simulink model "V.1.0.SystemsmModelling"  (R2020a)
settings: Solver=ode23t  StartTime=0.0  StopTime=2000  MaxStep=2000.0  RelTol=1e-3
values from neighbouring files (symbols this model uses):
  InitialTemp = 300    [Setup.m]
undefined symbols (not defined in the file or in its folder): commanded_mass_flow, compressor_time_constant, condenser_length, copper_density, environment_temperature, evaporator_length, ground_temperature, max_throat_area, max_throat_temperature, min_throat_area, min_throat_temperature, pipe_diameter, pipe_thickness, target_temperature, temperature_delta, u_sat
libraries: fl_lib x208, refrigeration_lib x90, fl_ps_legacy_lib x50, nesl_utility x45
(part 1 of 7)
settings Model: Creator=denni  LastModifiedBy=denni

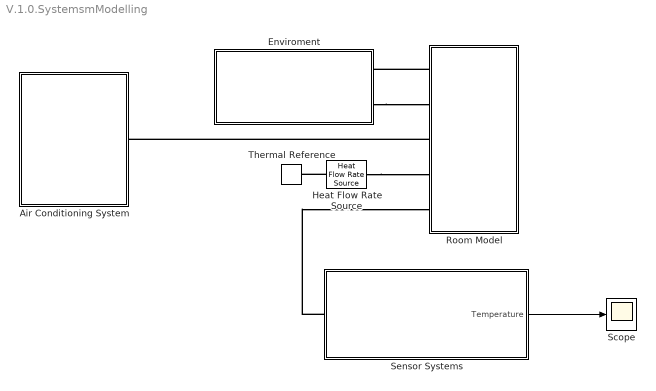
== system V.1.0.SystemsmModelling ==
  Air Conditioning System : Subsystem
  Enviroment : Subsystem
  Heat Flow Rate Source : fl_lib/Thermal/Thermal Sources/Heat Flow Rate Source  heat_flow=10 W
      settings: SourceProductBaseCode=SS  InternalSimscapePortConfiguration="{\"Bottom\":[],\"Left\":[{\"id\":\"B\",\"label\":\"B\",\"type\":\"foundation.thermal.thermal\"}],\"Right\":[{\"id\":\"A\",\"label\":\"A\",\"type\":\"foundation.thermal.thermal\"}],\"Top\":[]}"
  Room Model : Subsystem
  Scope : Scope
  Sensor Systems : Subsystem
  Thermal Reference : fl_lib/Thermal/Thermal Elements/Thermal Reference
  wires:
  Sensor Systems/1("Temperature ") -> Scope/1
  connections:
  Room Model/LConn1 -- Enviroment/LConn1
  Enviroment/LConn2 -- Room Model/LConn2
  Sensor Systems/LConn1 -- Room Model/LConn5
  Heat Flow Rate Source/LConn1 -- Room Model/LConn4
  Heat Flow Rate Source/RConn1 -- Thermal Reference/LConn1
  Room Model/LConn3 -- Air Conditioning System/RConn1

== system V.1.0.SystemsmModelling/Air Conditioning System ==
  Air Conditioner Model : Subsystem
  Air Conditioner Model1 : Subsystem
  Air Conditioner Model2 : Subsystem
  Air Conditioner Model3 : Subsystem
  Air Conditioner Model4 : Subsystem
  Air Conditioner Model5 : Subsystem
  Air Conditioner Model6 : Subsystem
  Air Conditioner Model7 : Subsystem
  Air Conditioner Model8 : Subsystem
  Air Conditioner Model9 : Subsystem
  Air : PMIOPort  Side=Right
  connections:
  Air Conditioner Model/LConn1 -- Air/RConn1 -- Air Conditioner Model1/LConn1 -- Air Conditioner Model2/LConn1 -- Air Conditioner Model5/LConn1 -- Air Conditioner Model8/LConn1 -- Air Conditioner Model9/LConn1 -- Air Conditioner Model7/LConn1 -- Air Conditioner Model6/LConn1 -- Air Conditioner Model4/LConn1 -- Air Conditioner Model3/LConn1

== system V.1.0.SystemsmModelling/Enviroment ==
  Atm Temperature Source : fl_lib/Thermal/Thermal Sources/Controlled Temperature Source
  Constant : Constant  Value=environment_temperature
  Constant1 : Constant  Value=ground_temperature
  Ground Temperature Source : fl_lib/Thermal/Thermal Sources/Controlled Temperature Source
  Simulink-PS Converter : nesl_utility/Simulink-PS Converter  PhysicalDomain=network_engine_domain  SubClassName=ps_input  LeftPortType=input  RightPortType=output  PseudoPeriodic=off  Frequencies=[]  NoiseDistribution=none  NoiseParameters=[]  Unit=1  AffineConversion=off  FilteringAndDerivatives=provide  SimscapeFilterOrder=1  InputFilterTimeConstant=0.001  UdotUserProvided=0
  Simulink-PS Converter1 : nesl_utility/Simulink-PS Converter  PhysicalDomain=network_engine_domain  SubClassName=ps_input  LeftPortType=input  RightPortType=output  PseudoPeriodic=off  Frequencies=[]  NoiseDistribution=none  NoiseParameters=[]  Unit=1  AffineConversion=off  FilteringAndDerivatives=provide  SimscapeFilterOrder=1  InputFilterTimeConstant=0.001  UdotUserProvided=0
  Thermal Reference1 : fl_lib/Thermal/Thermal Elements/Thermal Reference
  Thermal Reference2 : fl_lib/Thermal/Thermal Elements/Thermal Reference
  Atm Temperature Source1 : PMIOPort  Side=Left
  Ground Temperature Source1 : PMIOPort  Port=2  Side=Left
  wires:
  Constant/1 -> Simulink-PS Converter/1
  Constant1/1 -> Simulink-PS Converter1/1
  connections:
  Thermal Reference2/LConn1 -- Ground Temperature Source/RConn2
  Thermal Reference1/LConn1 -- Atm Temperature Source/RConn2
  Simulink-PS Converter1/RConn1 -- Ground Temperature Source/RConn1
  Ground Temperature Source/LConn1 -- Ground Temperature Source1/RConn1
  Atm Temperature Source1/RConn1 -- Atm Temperature Source/LConn1
  Simulink-PS Converter/RConn1 -- Atm Temperature Source/RConn1

== system V.1.0.SystemsmModelling/Room Model ==
  "Room Element " : Subsystem
  Solver Configuration : nesl_utility/Solver Configuration  PhysicalDomain=network_engine_domain  SubClassName=solver  LeftPortType=input  RightPortType=generic  Tones=[]  Harmonics=[]  SimulateNoise=off  Profile=off  UseLocalSampling=off  EnableSwitchedLinearOptims=on  FrequencyDomain=off  UseCCode=off  RelTol=0.001  AbsTol=1e-06  MinStep=1e-09  ToWorkspace=off  RevertToSquareIcSolve=off  NumHomotopyIterations=100  PhasorMode=off  PhasorModeNumHarmonics=1  DoDC=off  ResidualTolerance=1e-09  UseLocalSolver=off  LocalSolverChoice=NE_BACKWARD_EULER_ADVANCER  LocalSolverSampleTime=0.001  DoFixedCost=off  MaxNonlinIter=3  MaxModeIter=2  LinearAlgebra=auto  EquationFormulation=NE_TIME_EF  DelaysMemoryBudget=1024  AutomaticFiltering=on  FilteringTimeConstant=0.001  PartitionStorageMethod=AS_NEEDED  PartitionMemoryBudget=1024  PartitionMethod=ROBUST
  Thermal Mass Air : fl_lib/Thermal/Thermal Elements/Thermal Mass  mass=1 kg  sp_heat=1012 J/kg/K  T_specify=off  T_priority=High  T=300 K  T_nominal_specify=off  T_nominal_unit=K  T_nominal_value=1  Q_specify=off  Q_priority=None  Q=0 W  Q_nominal_specify=off  Q_nominal_unit=W  Q_nominal_value=1
  Atm-env : PMIOPort  Side=Left
  Ground-env : PMIOPort  Port=2  Side=Left
  Air Conditioner : PMIOPort  Port=3  Side=Left
  Server Racks : PMIOPort  Port=4  Side=Left
  "Room Temperature Sensor " : PMIOPort  Port=5  Side=Left
  connections:
  Thermal Mass Air/LConn1 -- Server Racks/RConn1 -- Air Conditioner/RConn1 -- "Room Temperature Sensor "/RConn1 -- Solver Configuration/RConn1 -- "Room Element "/LConn1
  Atm-env/RConn1 -- "Room Element "/LConn2
  "Room Element "/LConn3 -- Ground-env/RConn1

== system V.1.0.SystemsmModelling/Sensor Systems ==
  PS-Simulink Converter : nesl_utility/PS-Simulink Converter  PhysicalDomain=network_engine_domain  SubClassName=ps_output  LeftPortType=input  RightPortType=output  PseudoPeriodic=off  Frequencies=[]  Unit=inherit  AffineConversion=off
  Room Temperature Sensor : fl_lib/Thermal/Thermal Sensors/Temperature Sensor
  Thermal Reference : fl_lib/Thermal/Thermal Elements/Thermal Reference
  Room Temperature Sensor1 : PMIOPort  Side=Left
  "Temperature " : Outport
  wires:
  PS-Simulink Converter/1 -> "Temperature "/1
  connections:
  PS-Simulink Converter/LConn1 -- Room Temperature Sensor/RConn2
  Thermal Reference/LConn1 -- Room Temperature Sensor/RConn1
  Room Temperature Sensor/LConn1 -- Room Temperature Sensor1/RConn1

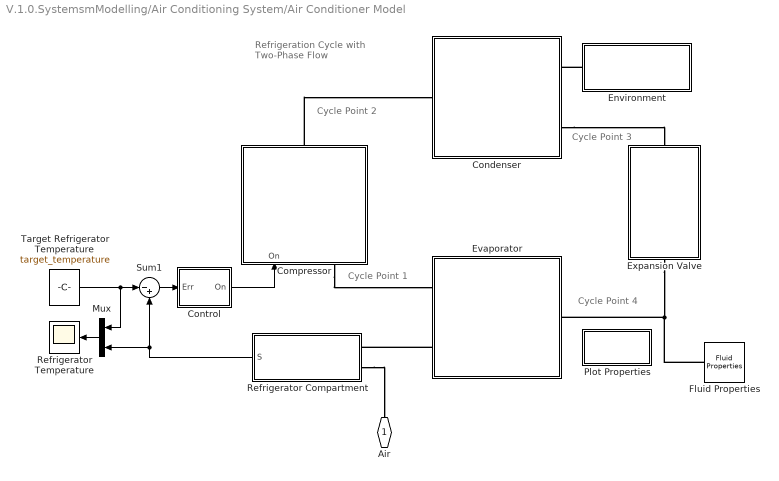
== system V.1.0.SystemsmModelling/Air Conditioning System/Air Conditioner Model ==
  note: Refrigeration Cycle
      | with Two-Phase Flow
  note: Cycle Point 1
  note: Cycle Point 3
  note: Cycle Point 2
  note: Cycle Point 4
  Compressor : Subsystem
      mask Display:
      | % Fading color
      | % Center to right
      | patch(sin(0.00*pi:0.05:1.10*pi),cos(0.00*pi:0.05:1.10*pi),[1;0.90;0.94]);
      | patch(sin(0.05*pi:0.05:0.95*pi),cos(0.05*pi:0.05:0.95*pi),[1;0.85;0.88]);
      | patch(sin(0.10*pi:0.05:0.90*pi),cos(0.10*pi:0.05:0.90*pi),[1;0.80;0.82]);
      | patch(sin(0.15*pi:0.05:0.85*pi),cos(0.15*pi:0.05:0.85*pi),[1;0.75;0.76]);
      | patch(sin(0.20*pi:0.05:0.80*pi),cos(0.20*pi:0.05:0.80*pi),[1;0.70;0.70]);
      | % Center to left
      | patch(sin(1.00*pi:0.05:2.00*pi),cos(1.00*pi:0.05:2.00*pi),[0.94;0.90;1]);
      | patch(sin(1.05*pi:0.05:1.95*pi),cos(1.05*pi:0.05:1.95*pi),[0.88;0.90;1]);
      | patch(sin(1.10*pi:0.05:1.90*pi),cos(1.10*pi:0.05:1.90*pi),[0.82;0.90;1]);
      | patch(sin(1.15*pi:0.05:1.85*pi),cos(1.15*pi:0.05:1.85*pi),[0.76;0.90;1]);
      | patch(sin(1.20*pi:0.05:1.80*pi),cos(1.20*pi:0.05:1.80*pi),[0.70;0.90;1]);
      | % Circle
      | plot(sin(0:0.1:2.2*pi),cos(0:0.1:2.2*pi));
      | % Angled lines
      | plot(sin([-0.6*pi/3 3.6*pi/8]),cos([-0.6*pi/3 3.6*pi/8]));
      | plot(sin([-0.6*pi/3 3.6*pi/8]),-cos([-0.6*pi/3 3.6*pi/8]));
      | plot(1.15*sin([-pi/4 3*pi/4]),1.15*cos([-pi/4 3*pi/4]));
      | % Arrow
      | patch([1.15*sin(-pi/4)+0.01;1.15*sin(3*pi/4)+0.01;1.15*sin(3*pi/4)-0.01;1.15*sin(-pi/4)-0.01],[1.15*cos(-pi/4)+0.01;1.15*cos(3*pi/4)+0.01;1.15*cos(3*pi/4)-0.01;1.15*cos(-pi/4)-0.01],[0;0;0])
      | patch([0.8*sin(3*pi/4)+0.05;1.15*sin(3*pi/4)+0.00;1.15*sin(3*pi/4)-0.00;0.8*sin(3*pi/4)-0.05],[0.8*cos(3*pi/4)+0.05;1.15*cos(3*pi/4)+0.00;1.15*cos(3*pi/4)-0.00;0.8*cos(3*pi/4)-0.05],[0;0;0])
      | % Points to set range for plotting area
      | color('white');plot(1.3,1.3);plot(-1.3,-1.3)
      | color('black');
      | 
      | port_label('LConn',1,'A');
      | port_label('RConn',1,'B');
      | port_label('input',1,'On');
  Condenser : Subsystem
      mask Display:
      | % Colored patches
      | % Center to right
      | patch(sin(0.0*pi:0.05:1.1*pi),cos(0.0*pi:0.05:1.1*pi),[1;0.58;0.58]);
      | patch(sin(0.1*pi:0.05:0.9*pi),cos(0.1*pi:0.05:0.9*pi),[1;0.64;0.64]);
      | patch(sin(0.2*pi:0.05:0.8*pi),cos(0.2*pi:0.05:0.8*pi),[1;0.70;0.70]);
      | % Center to left
      | patch(sin(1.0*pi:0.05:2.0*pi),cos(1.0*pi:0.05:2.0*pi),[1;0.52;0.52]);
      | patch(sin(1.1*pi:0.05:1.9*pi),cos(1.1*pi:0.05:1.9*pi),[1;0.46;0.46]);
      | patch(sin(1.2*pi:0.05:1.8*pi),cos(1.2*pi:0.05:1.8*pi),[1;0.40;0.40]);
      | % Circle
      | plot(sin(0:0.1:2.2*pi),cos(0:0.1:2.2*pi));
      | % 'M'
      | plot([0.5 0.5],[-1.2 0.5]);
      | plot([-0.5 -0.5],[-1.2 0.5]);
      | plot([0.5 0],[0.5 -0.2]);
      | plot([-0.5 0],[0.5 -0.2]);
      | % Plot points to set plot range
      | color('white');plot(1.3,1.3);plot(-1.3,-1.3)
      | color('black');
      | 
      | port_label('RConn',1,'A');
      | port_label('LConn',1,'T');
      | port_label('LConn',2,'B');
  Control : Subsystem
  Environment : Subsystem
      mask Display:
      | % Colored patch
      | patch([sin(0:0.1:1*pi)*0.25+0.4 sin(pi:0.1:2*pi)*0.25-0.4],[cos(0:0.1:1*pi) cos(pi:0.1:2*pi)],[1;0.9;0.9]);
      | % Outer rounded rectangle
      | plot(sin(0:0.1:1*pi)*0.25+0.4,cos(0:0.1:1*pi));
      | plot(sin(pi:0.1:2*pi)*0.25-0.4,cos(pi:0.1:2*pi));
      | plot([-0.4 0.4],[1 1]);
      | plot([-0.4 0.4],[-1 -1]);
      | % House frame
      | plot([-0.3 -0.3],[-0.866,0.866*0.2])
      | plot([0.3 0.3],[-0.866,0.866*0.2])
      | plot([0.3 0],[0.866*0.2, 0.866])
      | plot([-0.3 0],[0.866*0.2, 0.866])
      | plot([-0.3 0.3],[-0.866 -0.866])
      | plot([-0.3 0.3],[0.866 0.866]*0.2)
      | plot([-0.2 -0.04],[0.866 0.866]*0)
      | % Window
      | plot([-0.2 -0.04],[-1 -1]*0.2)
      | plot([-0.2 -0.04],[-1 -1]*0.4)
      | plot([-0.2 -0.2],[0 -0.4])
      | plot([-0.12 -0.12],[0 -0.4])
      | plot([-0.04 -0.04],[0 -0.4])
      | % Door
      | plot([0.05 0.05],[-0.866 -0.2])
      | plot([0.18 0.18],[-0.866 -0.2])
      | plot([0.05 0.18],[-0.2 -0.2])
      | patch([0.12 0.15 0.12 0.15],[-0.5 -0.5 -0.54 -0.54],[0;0;0])
      | % Outer boundary (so plot labels are visible)
      | color('white');plot(0.8660,0.8660);plot(-0.8660,-0.8660)
      | color('black');
      | port_label('LConn',1,'T');
  Evaporator : Subsystem
      mask Display:
      | % Fading color
      | % Center to right
      | patch(sin(0.00*pi:0.05:1.10*pi),cos(0.00*pi:0.05:1.10*pi),[0.58;0.70;1]);
      | patch(sin(0.05*pi:0.05:0.95*pi),cos(0.05*pi:0.05:0.95*pi),[0.63;0.75;1]);
      | patch(sin(0.10*pi:0.05:0.90*pi),cos(0.10*pi:0.05:0.90*pi),[0.66;0.80;1]);
      | patch(sin(0.15*pi:0.05:0.85*pi),cos(0.15*pi:0.05:0.85*pi),[0.69;0.85;1]);
      | patch(sin(0.20*pi:0.05:0.80*pi),cos(0.20*pi:0.05:0.80*pi),[0.70;0.90;1]);
      | % Center to left
      | patch(sin(1.00*pi:0.05:2.00*pi),cos(1.00*pi:0.05:2.00*pi),[0.52;0.60;1]);
      | patch(sin(1.05*pi:0.05:1.95*pi),cos(1.05*pi:0.05:1.95*pi),[0.49;0.55;1]);
      | patch(sin(1.10*pi:0.05:1.90*pi),cos(1.10*pi:0.05:1.90*pi),[0.46;0.50;1]);
      | patch(sin(1.15*pi:0.05:1.85*pi),cos(1.15*pi:0.05:1.85*pi),[0.43;0.45;1]);
      | patch(sin(1.20*pi:0.05:1.80*pi),cos(1.20*pi:0.05:1.80*pi),[0.40;0.40;1]);
      | % Circle
      | plot(sin(0:0.1:2.2*pi),cos(0:0.1:2.2*pi));
      | % 'M'
      | plot([0.5 0.5],[-1.2 0.5]);
      | plot([-0.5 -0.5],[-1.2 0.5]);
      | plot([0.5 0],[0.5 -0.2]);
      | plot([-0.5 0],[0.5 -0.2]);
      | % Plot points to set plotting range
      | color('white');plot(1.3,1.3);plot(-1.3,-1.3)
      | color('black');
      | 
      | port_label('LConn',1,'A');
      | port_label('RConn',1,'B');
      | port_label('RConn',2,'T');
  Expansion Valve : Subsystem
      mask Display:
      | % Colored patches
      | patch([-1 -1 0],[0.5 -0.5 0],[1;0.4;0.4]);
      | patch([1 1 0],[0.5 -0.5 0],[0.4;0.4;1]);
      | % Valve
      | plot([1 1],[0.5 -0.5]);
      | plot([-1 -1],[0.5 -0.5]);
      | plot([-1 1],[0.5 -0.5]);
      | plot([-1 1],[-0.5 0.5]);
      | % Arrow
      | patch([1.15*sin(-pi/4-0.01);1.15*sin(-pi/4+0.01);1*sin(3*pi/4-0.01);1*sin(3*pi/4+0.01)],[1.15*cos(-pi/4-0.01);1.15*cos(-pi/4+0.01);1*cos(3*pi/4-0.01);1*cos(3*pi/4+0.01)],[0;0;0])
      | patch([0.8*sin(3*pi/4+0.07);1.15*sin(3*pi/4+0.00);1.15*sin(3*pi/4-0.00);0.8*sin(3*pi/4-0.07)],[0.8*cos(3*pi/4+0.07);1.15*cos(3*pi/4+0.00);1.15*cos(3*pi/4-0.00);0.8*cos(3*pi/4-0.07)],[0;0;0])
      | % Plot outer points to set plot range
      | color('white'); plot(-1.3,0); plot(1.3,0);
      | color('black');
      | port_label('LConn',1,'A');
      | port_label('RConn',1,'B');
  Fluid Properties : refrigeration_lib/Fluid Properties  p_TLU=p_TLU MPa  u_TLU=u_TLU kJ/kg  v_TLU=v_TLU m^3/kg  T_TLU=T_TLU K  mu_TLU=mu_TLU s*uPa  k_TLU=k_TLU W/(m*K)  Pr_TLU=Pr_TLU  u_liq=u_sat(:,1) kJ/kg  u_vap=u_sat(:,2) kJ/kg
      settings: InternalSimscapePortConfiguration="{\"Bottom\":[],\"Left\":[],\"Right\":[{\"id\":\"A\",\"label\":\"\",\"type\":\"refrigeration.refrigeration\"}],\"Top\":[]}"
  Mux : Mux  Inputs=2
  Plot Properties : Subsystem
      settings: OpenFcn=plotFluidProperties()
      mask Display: disp('Plot Fluid\nProperties');
  Refrigerator Compartment : Subsystem
      mask Display:
      | % Color
      | patch([sin(0:0.1:1*pi)*0.25+0.4 sin(pi:0.1:2*pi)*0.25-0.4],[cos(0:0.1:1*pi) cos(pi:0.1:2*pi)],[0.70;0.90;1]);
      | % Outer rounded rectangle
      | plot(sin(pi:0.1:2*pi)*0.25-0.4,cos(pi:0.1:2*pi));
      | plot(sin(0:0.1:1*pi)*0.25+0.4,cos(0:0.1:1*pi));
      | plot(sin(pi:0.1:2*pi)*0.25-0.4,cos(pi:0.1:2*pi));
      | plot([-0.4 0.4],[1 1]);
      | plot([-0.4 0.4],[-1 -1]);
      | % Outer points to set size of plot range
      | color('white');plot(0.8660,0.8660);plot(-0.8660,-0.8660)
      | color('black');
      | % Snowflake
      | plot([0 0],[0.8 -0.8]);
      | plot([0 0.1],[0.5 0.7]);
      | plot([0 -0.1],[0.5 0.7]);
      | plot([0 0.1],[-0.5 -0.7]);
      | plot([0 -0.1],[-0.5 -0.7]);
      | plot(0.3*sin([pi/3 4*pi/3]),1*cos([pi/3 4*pi/3]));
      | plot([0.22*sin(pi/3) 0.25*sin(pi/4)],[0.7*cos(pi/3) 0.84*cos(pi/4)]);
      | plot([0.22*sin(pi/3) 0.25*sin(pi/2)],[0.7*cos(pi/3) 0.325*cos(pi/4)]);
      | plot([0.22*sin(pi/3) 0.25*sin(pi/4)],[-0.7*cos(pi/3) -0.84*cos(pi/4)]);
      | plot([0.22*sin(pi/3) 0.25*sin(pi/2)],[-0.7*cos(pi/3) -0.325*cos(pi/4)]);
      | plot(-0.3*sin([pi/3 4*pi/3]),1*cos([pi/3 4*pi/3]));
      | plot([-0.22*sin(pi/3) -0.25*sin(pi/4)],[0.7*cos(pi/3) 0.84*cos(pi/4)]);
      | plot([-0.22*sin(pi/3) -0.25*sin(pi/2)],[0.7*cos(pi/3) 0.325*cos(pi/4)]);
      | plot([-0.22*sin(pi/3) -0.25*sin(pi/4)],[-0.7*cos(pi/3) -0.84*cos(pi/4)]);
      | plot([-0.22*sin(pi/3) -0.25*sin(pi/2)],[-0.7*cos(pi/3) -0.325*cos(pi/4)]);
      | plot([0 0.1],[-0.5 -0.7]);
      | plot([0 -0.1],[-0.5 -0.7]);
      | % Labels
      | port_label('LConn',1,'T');
      | port_label('output',1,'S');
  Refrigerator Temperature : Scope
  Sum1 : Sum  Inputs=|-+
  Target Refrigerator Temperature : Constant  Value=target_temperature
  Air : PMIOPort  Side=Left
  wires:
  Control/1(On) -> Compressor/1(On)
  Refrigerator Compartment/1(S) -> Mux/2, Sum1/2
  Target Refrigerator Temperature/1 -> Sum1/1, Mux/1
  Mux/1 -> Refrigerator Temperature/1
  Sum1/1 -> Control/1(Err)
  connections:
  Expansion Valve/RConn1 -- Fluid Properties/RConn1 -- Evaporator/LConn1
  Environment/LConn1 -- Condenser/LConn1
  Evaporator/RConn2 -- Refrigerator Compartment/LConn1
  Compressor/LConn1 -- Evaporator/RConn1
  Condenser/LConn2 -- Expansion Valve/LConn1
  Compressor/RConn1 -- Condenser/RConn1
  Refrigerator Compartment/LConn2 -- Air/RConn1

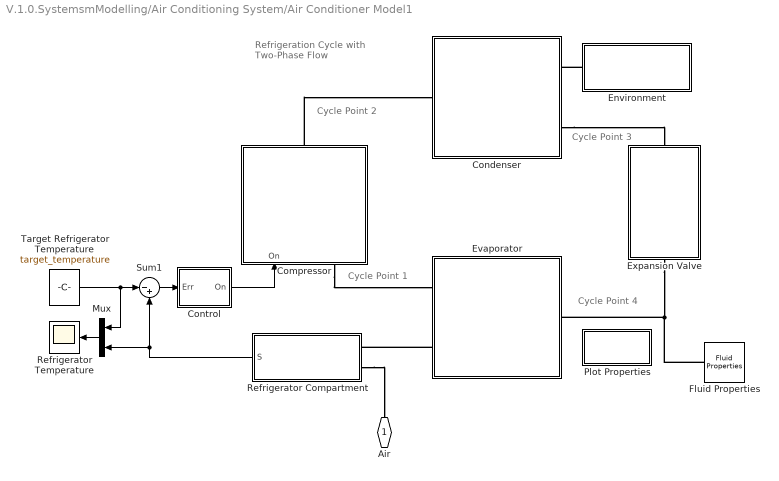
== system V.1.0.SystemsmModelling/Air Conditioning System/Air Conditioner Model1 ==
  note: Refrigeration Cycle
      | with Two-Phase Flow
  note: Cycle Point 1
  note: Cycle Point 3
  note: Cycle Point 2
  note: Cycle Point 4
  Compressor : Subsystem
      mask Display:
      | % Fading color
      | % Center to right
      | patch(sin(0.00*pi:0.05:1.10*pi),cos(0.00*pi:0.05:1.10*pi),[1;0.90;0.94]);
      | patch(sin(0.05*pi:0.05:0.95*pi),cos(0.05*pi:0.05:0.95*pi),[1;0.85;0.88]);
      | patch(sin(0.10*pi:0.05:0.90*pi),cos(0.10*pi:0.05:0.90*pi),[1;0.80;0.82]);
      | patch(sin(0.15*pi:0.05:0.85*pi),cos(0.15*pi:0.05:0.85*pi),[1;0.75;0.76]);
      | patch(sin(0.20*pi:0.05:0.80*pi),cos(0.20*pi:0.05:0.80*pi),[1;0.70;0.70]);
      | % Center to left
      | patch(sin(1.00*pi:0.05:2.00*pi),cos(1.00*pi:0.05:2.00*pi),[0.94;0.90;1]);
      | patch(sin(1.05*pi:0.05:1.95*pi),cos(1.05*pi:0.05:1.95*pi),[0.88;0.90;1]);
      | patch(sin(1.10*pi:0.05:1.90*pi),cos(1.10*pi:0.05:1.90*pi),[0.82;0.90;1]);
      | patch(sin(1.15*pi:0.05:1.85*pi),cos(1.15*pi:0.05:1.85*pi),[0.76;0.90;1]);
      | patch(sin(1.20*pi:0.05:1.80*pi),cos(1.20*pi:0.05:1.80*pi),[0.70;0.90;1]);
      | % Circle
      | plot(sin(0:0.1:2.2*pi),cos(0:0.1:2.2*pi));
      | % Angled lines
      | plot(sin([-0.6*pi/3 3.6*pi/8]),cos([-0.6*pi/3 3.6*pi/8]));
      | plot(sin([-0.6*pi/3 3.6*pi/8]),-cos([-0.6*pi/3 3.6*pi/8]));
      | plot(1.15*sin([-pi/4 3*pi/4]),1.15*cos([-pi/4 3*pi/4]));
      | % Arrow
      | patch([1.15*sin(-pi/4)+0.01;1.15*sin(3*pi/4)+0.01;1.15*sin(3*pi/4)-0.01;1.15*sin(-pi/4)-0.01],[1.15*cos(-pi/4)+0.01;1.15*cos(3*pi/4)+0.01;1.15*cos(3*pi/4)-0.01;1.15*cos(-pi/4)-0.01],[0;0;0])
      | patch([0.8*sin(3*pi/4)+0.05;1.15*sin(3*pi/4)+0.00;1.15*sin(3*pi/4)-0.00;0.8*sin(3*pi/4)-0.05],[0.8*cos(3*pi/4)+0.05;1.15*cos(3*pi/4)+0.00;1.15*cos(3*pi/4)-0.00;0.8*cos(3*pi/4)-0.05],[0;0;0])
      | % Points to set range for plotting area
      | color('white');plot(1.3,1.3);plot(-1.3,-1.3)
      | color('black');
      | 
      | port_label('LConn',1,'A');
      | port_label('RConn',1,'B');
      | port_label('input',1,'On');
  Condenser : Subsystem
      mask Display:
      | % Colored patches
      | % Center to right
      | patch(sin(0.0*pi:0.05:1.1*pi),cos(0.0*pi:0.05:1.1*pi),[1;0.58;0.58]);
      | patch(sin(0.1*pi:0.05:0.9*pi),cos(0.1*pi:0.05:0.9*pi),[1;0.64;0.64]);
      | patch(sin(0.2*pi:0.05:0.8*pi),cos(0.2*pi:0.05:0.8*pi),[1;0.70;0.70]);
      | % Center to left
      | patch(sin(1.0*pi:0.05:2.0*pi),cos(1.0*pi:0.05:2.0*pi),[1;0.52;0.52]);
      | patch(sin(1.1*pi:0.05:1.9*pi),cos(1.1*pi:0.05:1.9*pi),[1;0.46;0.46]);
      | patch(sin(1.2*pi:0.05:1.8*pi),cos(1.2*pi:0.05:1.8*pi),[1;0.40;0.40]);
      | % Circle
      | plot(sin(0:0.1:2.2*pi),cos(0:0.1:2.2*pi));
      | % 'M'
      | plot([0.5 0.5],[-1.2 0.5]);
      | plot([-0.5 -0.5],[-1.2 0.5]);
      | plot([0.5 0],[0.5 -0.2]);
      | plot([-0.5 0],[0.5 -0.2]);
      | % Plot points to set plot range
      | color('white');plot(1.3,1.3);plot(-1.3,-1.3)
      | color('black');
      | 
      | port_label('RConn',1,'A');
      | port_label('LConn',1,'T');
      | port_label('LConn',2,'B');
  Control : Subsystem
  Environment : Subsystem
      mask Display:
      | % Colored patch
      | patch([sin(0:0.1:1*pi)*0.25+0.4 sin(pi:0.1:2*pi)*0.25-0.4],[cos(0:0.1:1*pi) cos(pi:0.1:2*pi)],[1;0.9;0.9]);
      | % Outer rounded rectangle
      | plot(sin(0:0.1:1*pi)*0.25+0.4,cos(0:0.1:1*pi));
      | plot(sin(pi:0.1:2*pi)*0.25-0.4,cos(pi:0.1:2*pi));
      | plot([-0.4 0.4],[1 1]);
      | plot([-0.4 0.4],[-1 -1]);
      | % House frame
      | plot([-0.3 -0.3],[-0.866,0.866*0.2])
      | plot([0.3 0.3],[-0.866,0.866*0.2])
      | plot([0.3 0],[0.866*0.2, 0.866])
      | plot([-0.3 0],[0.866*0.2, 0.866])
      | plot([-0.3 0.3],[-0.866 -0.866])
      | plot([-0.3 0.3],[0.866 0.866]*0.2)
      | plot([-0.2 -0.04],[0.866 0.866]*0)
      | % Window
      | plot([-0.2 -0.04],[-1 -1]*0.2)
      | plot([-0.2 -0.04],[-1 -1]*0.4)
      | plot([-0.2 -0.2],[0 -0.4])
      | plot([-0.12 -0.12],[0 -0.4])
      | plot([-0.04 -0.04],[0 -0.4])
      | % Door
      | plot([0.05 0.05],[-0.866 -0.2])
      | plot([0.18 0.18],[-0.866 -0.2])
      | plot([0.05 0.18],[-0.2 -0.2])
      | patch([0.12 0.15 0.12 0.15],[-0.5 -0.5 -0.54 -0.54],[0;0;0])
      | % Outer boundary (so plot labels are visible)
      | color('white');plot(0.8660,0.8660);plot(-0.8660,-0.8660)
      | color('black');
      | port_label('LConn',1,'T');
  Evaporator : Subsystem
      mask Display:
      | % Fading color
      | % Center to right
      | patch(sin(0.00*pi:0.05:1.10*pi),cos(0.00*pi:0.05:1.10*pi),[0.58;0.70;1]);
      | patch(sin(0.05*pi:0.05:0.95*pi),cos(0.05*pi:0.05:0.95*pi),[0.63;0.75;1]);
      | patch(sin(0.10*pi:0.05:0.90*pi),cos(0.10*pi:0.05:0.90*pi),[0.66;0.80;1]);
      | patch(sin(0.15*pi:0.05:0.85*pi),cos(0.15*pi:0.05:0.85*pi),[0.69;0.85;1]);
      | patch(sin(0.20*pi:0.05:0.80*pi),cos(0.20*pi:0.05:0.80*pi),[0.70;0.90;1]);
      | % Center to left
      | patch(sin(1.00*pi:0.05:2.00*pi),cos(1.00*pi:0.05:2.00*pi),[0.52;0.60;1]);
      | patch(sin(1.05*pi:0.05:1.95*pi),cos(1.05*pi:0.05:1.95*pi),[0.49;0.55;1]);
      | patch(sin(1.10*pi:0.05:1.90*pi),cos(1.10*pi:0.05:1.90*pi),[0.46;0.50;1]);
      | patch(sin(1.15*pi:0.05:1.85*pi),cos(1.15*pi:0.05:1.85*pi),[0.43;0.45;1]);
      | patch(sin(1.20*pi:0.05:1.80*pi),cos(1.20*pi:0.05:1.80*pi),[0.40;0.40;1]);
      | % Circle
      | plot(sin(0:0.1:2.2*pi),cos(0:0.1:2.2*pi));
      | % 'M'
      | plot([0.5 0.5],[-1.2 0.5]);
      | plot([-0.5 -0.5],[-1.2 0.5]);
      | plot([0.5 0],[0.5 -0.2]);
      | plot([-0.5 0],[0.5 -0.2]);
      | % Plot points to set plotting range
      | color('white');plot(1.3,1.3);plot(-1.3,-1.3)
      | color('black');
      | 
      | port_label('LConn',1,'A');
      | port_label('RConn',1,'B');
      | port_label('RConn',2,'T');
  Expansion Valve : Subsystem
      mask Display:
      | % Colored patches
      | patch([-1 -1 0],[0.5 -0.5 0],[1;0.4;0.4]);
      | patch([1 1 0],[0.5 -0.5 0],[0.4;0.4;1]);
      | % Valve
      | plot([1 1],[0.5 -0.5]);
      | plot([-1 -1],[0.5 -0.5]);
      | plot([-1 1],[0.5 -0.5]);
      | plot([-1 1],[-0.5 0.5]);
      | % Arrow
      | patch([1.15*sin(-pi/4-0.01);1.15*sin(-pi/4+0.01);1*sin(3*pi/4-0.01);1*sin(3*pi/4+0.01)],[1.15*cos(-pi/4-0.01);1.15*cos(-pi/4+0.01);1*cos(3*pi/4-0.01);1*cos(3*pi/4+0.01)],[0;0;0])
      | patch([0.8*sin(3*pi/4+0.07);1.15*sin(3*pi/4+0.00);1.15*sin(3*pi/4-0.00);0.8*sin(3*pi/4-0.07)],[0.8*cos(3*pi/4+0.07);1.15*cos(3*pi/4+0.00);1.15*cos(3*pi/4-0.00);0.8*cos(3*pi/4-0.07)],[0;0;0])
      | % Plot outer points to set plot range
      | color('white'); plot(-1.3,0); plot(1.3,0);
      | color('black');
      | port_label('LConn',1,'A');
      | port_label('RConn',1,'B');
  Fluid Properties : refrigeration_lib/Fluid Properties  p_TLU=p_TLU MPa  u_TLU=u_TLU kJ/kg  v_TLU=v_TLU m^3/kg  T_TLU=T_TLU K  mu_TLU=mu_TLU s*uPa  k_TLU=k_TLU W/(m*K)  Pr_TLU=Pr_TLU  u_liq=u_sat(:,1) kJ/kg  u_vap=u_sat(:,2) kJ/kg
      settings: InternalSimscapePortConfiguration="{\"Bottom\":[],\"Left\":[],\"Right\":[{\"id\":\"A\",\"label\":\"\",\"type\":\"refrigeration.refrigeration\"}],\"Top\":[]}"
  Mux : Mux  Inputs=2
  Plot Properties : Subsystem
      settings: OpenFcn=plotFluidProperties()
      mask Display: disp('Plot Fluid\nProperties');
  Refrigerator Compartment : Subsystem
      mask Display:
      | % Color
      | patch([sin(0:0.1:1*pi)*0.25+0.4 sin(pi:0.1:2*pi)*0.25-0.4],[cos(0:0.1:1*pi) cos(pi:0.1:2*pi)],[0.70;0.90;1]);
      | % Outer rounded rectangle
      | plot(sin(pi:0.1:2*pi)*0.25-0.4,cos(pi:0.1:2*pi));
      | plot(sin(0:0.1:1*pi)*0.25+0.4,cos(0:0.1:1*pi));
      | plot(sin(pi:0.1:2*pi)*0.25-0.4,cos(pi:0.1:2*pi));
      | plot([-0.4 0.4],[1 1]);
      | plot([-0.4 0.4],[-1 -1]);
      | % Outer points to set size of plot range
      | color('white');plot(0.8660,0.8660);plot(-0.8660,-0.8660)
      | color('black');
      | % Snowflake
      | plot([0 0],[0.8 -0.8]);
      | plot([0 0.1],[0.5 0.7]);
      | plot([0 -0.1],[0.5 0.7]);
      | plot([0 0.1],[-0.5 -0.7]);
      | plot([0 -0.1],[-0.5 -0.7]);
      | plot(0.3*sin([pi/3 4*pi/3]),1*cos([pi/3 4*pi/3]));
      | plot([0.22*sin(pi/3) 0.25*sin(pi/4)],[0.7*cos(pi/3) 0.84*cos(pi/4)]);
      | plot([0.22*sin(pi/3) 0.25*sin(pi/2)],[0.7*cos(pi/3) 0.325*cos(pi/4)]);
      | plot([0.22*sin(pi/3) 0.25*sin(pi/4)],[-0.7*cos(pi/3) -0.84*cos(pi/4)]);
      | plot([0.22*sin(pi/3) 0.25*sin(pi/2)],[-0.7*cos(pi/3) -0.325*cos(pi/4)]);
      | plot(-0.3*sin([pi/3 4*pi/3]),1*cos([pi/3 4*pi/3]));
      | plot([-0.22*sin(pi/3) -0.25*sin(pi/4)],[0.7*cos(pi/3) 0.84*cos(pi/4)]);
      | plot([-0.22*sin(pi/3) -0.25*sin(pi/2)],[0.7*cos(pi/3) 0.325*cos(pi/4)]);
      | plot([-0.22*sin(pi/3) -0.25*sin(pi/4)],[-0.7*cos(pi/3) -0.84*cos(pi/4)]);
      | plot([-0.22*sin(pi/3) -0.25*sin(pi/2)],[-0.7*cos(pi/3) -0.325*cos(pi/4)]);
      | plot([0 0.1],[-0.5 -0.7]);
      | plot([0 -0.1],[-0.5 -0.7]);
      | % Labels
      | port_label('LConn',1,'T');
      | port_label('output',1,'S');
  Refrigerator Temperature : Scope
  Sum1 : Sum  Inputs=|-+
  Target Refrigerator Temperature : Constant  Value=target_temperature
  Air : PMIOPort  Side=Left
  wires:
  Control/1(On) -> Compressor/1(On)
  Refrigerator Compartment/1(S) -> Mux/2, Sum1/2
  Target Refrigerator Temperature/1 -> Sum1/1, Mux/1
  Mux/1 -> Refrigerator Temperature/1
  Sum1/1 -> Control/1(Err)
  connections:
  Expansion Valve/RConn1 -- Fluid Properties/RConn1 -- Evaporator/LConn1
  Environment/LConn1 -- Condenser/LConn1
  Evaporator/RConn2 -- Refrigerator Compartment/LConn1
  Compressor/LConn1 -- Evaporator/RConn1
  Condenser/LConn2 -- Expansion Valve/LConn1
  Compressor/RConn1 -- Condenser/RConn1
  Refrigerator Compartment/LConn2 -- Air/RConn1

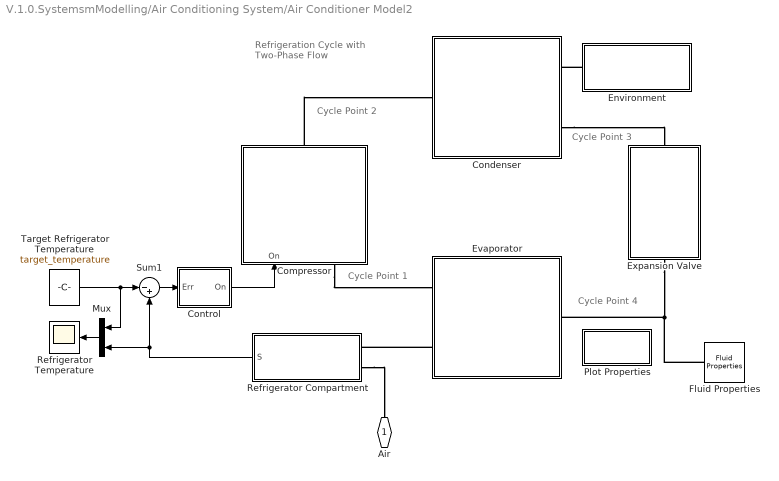
== system V.1.0.SystemsmModelling/Air Conditioning System/Air Conditioner Model2 ==
  note: Refrigeration Cycle
      | with Two-Phase Flow
  note: Cycle Point 1
  note: Cycle Point 3
  note: Cycle Point 2
  note: Cycle Point 4
  Compressor : Subsystem
      mask Display:
      | % Fading color
      | % Center to right
      | patch(sin(0.00*pi:0.05:1.10*pi),cos(0.00*pi:0.05:1.10*pi),[1;0.90;0.94]);
      | patch(sin(0.05*pi:0.05:0.95*pi),cos(0.05*pi:0.05:0.95*pi),[1;0.85;0.88]);
      | patch(sin(0.10*pi:0.05:0.90*pi),cos(0.10*pi:0.05:0.90*pi),[1;0.80;0.82]);
      | patch(sin(0.15*pi:0.05:0.85*pi),cos(0.15*pi:0.05:0.85*pi),[1;0.75;0.76]);
      | patch(sin(0.20*pi:0.05:0.80*pi),cos(0.20*pi:0.05:0.80*pi),[1;0.70;0.70]);
      | % Center to left
      | patch(sin(1.00*pi:0.05:2.00*pi),cos(1.00*pi:0.05:2.00*pi),[0.94;0.90;1]);
      | patch(sin(1.05*pi:0.05:1.95*pi),cos(1.05*pi:0.05:1.95*pi),[0.88;0.90;1]);
      | patch(sin(1.10*pi:0.05:1.90*pi),cos(1.10*pi:0.05:1.90*pi),[0.82;0.90;1]);
      | patch(sin(1.15*pi:0.05:1.85*pi),cos(1.15*pi:0.05:1.85*pi),[0.76;0.90;1]);
      | patch(sin(1.20*pi:0.05:1.80*pi),cos(1.20*pi:0.05:1.80*pi),[0.70;0.90;1]);
      | % Circle
      | plot(sin(0:0.1:2.2*pi),cos(0:0.1:2.2*pi));
      | % Angled lines
      | plot(sin([-0.6*pi/3 3.6*pi/8]),cos([-0.6*pi/3 3.6*pi/8]));
      | plot(sin([-0.6*pi/3 3.6*pi/8]),-cos([-0.6*pi/3 3.6*pi/8]));
      | plot(1.15*sin([-pi/4 3*pi/4]),1.15*cos([-pi/4 3*pi/4]));
      | % Arrow
      | patch([1.15*sin(-pi/4)+0.01;1.15*sin(3*pi/4)+0.01;1.15*sin(3*pi/4)-0.01;1.15*sin(-pi/4)-0.01],[1.15*cos(-pi/4)+0.01;1.15*cos(3*pi/4)+0.01;1.15*cos(3*pi/4)-0.01;1.15*cos(-pi/4)-0.01],[0;0;0])
      | patch([0.8*sin(3*pi/4)+0.05;1.15*sin(3*pi/4)+0.00;1.15*sin(3*pi/4)-0.00;0.8*sin(3*pi/4)-0.05],[0.8*cos(3*pi/4)+0.05;1.15*cos(3*pi/4)+0.00;1.15*cos(3*pi/4)-0.00;0.8*cos(3*pi/4)-0.05],[0;0;0])
      | % Points to set range for plotting area
      | color('white');plot(1.3,1.3);plot(-1.3,-1.3)
      | color('black');
      | 
      | port_label('LConn',1,'A');
      | port_label('RConn',1,'B');
      | port_label('input',1,'On');
  Condenser : Subsystem
      mask Display:
      | % Colored patches
      | % Center to right
      | patch(sin(0.0*pi:0.05:1.1*pi),cos(0.0*pi:0.05:1.1*pi),[1;0.58;0.58]);
      | patch(sin(0.1*pi:0.05:0.9*pi),cos(0.1*pi:0.05:0.9*pi),[1;0.64;0.64]);
      | patch(sin(0.2*pi:0.05:0.8*pi),cos(0.2*pi:0.05:0.8*pi),[1;0.70;0.70]);
      | % Center to left
      | patch(sin(1.0*pi:0.05:2.0*pi),cos(1.0*pi:0.05:2.0*pi),[1;0.52;0.52]);
      | patch(sin(1.1*pi:0.05:1.9*pi),cos(1.1*pi:0.05:1.9*pi),[1;0.46;0.46]);
      | patch(sin(1.2*pi:0.05:1.8*pi),cos(1.2*pi:0.05:1.8*pi),[1;0.40;0.40]);
      | % Circle
      | plot(sin(0:0.1:2.2*pi),cos(0:0.1:2.2*pi));
      | % 'M'
      | plot([0.5 0.5],[-1.2 0.5]);
      | plot([-0.5 -0.5],[-1.2 0.5]);
      | plot([0.5 0],[0.5 -0.2]);
      | plot([-0.5 0],[0.5 -0.2]);
      | % Plot points to set plot range
      | color('white');plot(1.3,1.3);plot(-1.3,-1.3)
      | color('black');
      | 
      | port_label('RConn',1,'A');
      | port_label('LConn',1,'T');
      | port_label('LConn',2,'B');
  Control : Subsystem
  Environment : Subsystem
      mask Display:
      | % Colored patch
      | patch([sin(0:0.1:1*pi)*0.25+0.4 sin(pi:0.1:2*pi)*0.25-0.4],[cos(0:0.1:1*pi) cos(pi:0.1:2*pi)],[1;0.9;0.9]);
      | % Outer rounded rectangle
      | plot(sin(0:0.1:1*pi)*0.25+0.4,cos(0:0.1:1*pi));
      | plot(sin(pi:0.1:2*pi)*0.25-0.4,cos(pi:0.1:2*pi));
      | plot([-0.4 0.4],[1 1]);
      | plot([-0.4 0.4],[-1 -1]);
      | % House frame
      | plot([-0.3 -0.3],[-0.866,0.866*0.2])
      | plot([0.3 0.3],[-0.866,0.866*0.2])
      | plot([0.3 0],[0.866*0.2, 0.866])
      | plot([-0.3 0],[0.866*0.2, 0.866])
      | plot([-0.3 0.3],[-0.866 -0.866])
      | plot([-0.3 0.3],[0.866 0.866]*0.2)
      | plot([-0.2 -0.04],[0.866 0.866]*0)
      | % Window
      | plot([-0.2 -0.04],[-1 -1]*0.2)
      | plot([-0.2 -0.04],[-1 -1]*0.4)
      | plot([-0.2 -0.2],[0 -0.4])
      | plot([-0.12 -0.12],[0 -0.4])
      | plot([-0.04 -0.04],[0 -0.4])
      | % Door
      | plot([0.05 0.05],[-0.866 -0.2])
      | plot([0.18 0.18],[-0.866 -0.2])
      | plot([0.05 0.18],[-0.2 -0.2])
      | patch([0.12 0.15 0.12 0.15],[-0.5 -0.5 -0.54 -0.54],[0;0;0])
      | % Outer boundary (so plot labels are visible)
      | color('white');plot(0.8660,0.8660);plot(-0.8660,-0.8660)
      | color('black');
      | port_label('LConn',1,'T');
  Evaporator : Subsystem
      mask Display:
      | % Fading color
      | % Center to right
      | patch(sin(0.00*pi:0.05:1.10*pi),cos(0.00*pi:0.05:1.10*pi),[0.58;0.70;1]);
      | patch(sin(0.05*pi:0.05:0.95*pi),cos(0.05*pi:0.05:0.95*pi),[0.63;0.75;1]);
      | patch(sin(0.10*pi:0.05:0.90*pi),cos(0.10*pi:0.05:0.90*pi),[0.66;0.80;1]);
      | patch(sin(0.15*pi:0.05:0.85*pi),cos(0.15*pi:0.05:0.85*pi),[0.69;0.85;1]);
      | patch(sin(0.20*pi:0.05:0.80*pi),cos(0.20*pi:0.05:0.80*pi),[0.70;0.90;1]);
      | % Center to left
      | patch(sin(1.00*pi:0.05:2.00*pi),cos(1.00*pi:0.05:2.00*pi),[0.52;0.60;1]);
      | patch(sin(1.05*pi:0.05:1.95*pi),cos(1.05*pi:0.05:1.95*pi),[0.49;0.55;1]);
      | patch(sin(1.10*pi:0.05:1.90*pi),cos(1.10*pi:0.05:1.90*pi),[0.46;0.50;1]);
      | patch(sin(1.15*pi:0.05:1.85*pi),cos(1.15*pi:0.05:1.85*pi),[0.43;0.45;1]);
      | patch(sin(1.20*pi:0.05:1.80*pi),cos(1.20*pi:0.05:1.80*pi),[0.40;0.40;1]);
      | % Circle
      | plot(sin(0:0.1:2.2*pi),cos(0:0.1:2.2*pi));
      | % 'M'
      | plot([0.5 0.5],[-1.2 0.5]);
      | plot([-0.5 -0.5],[-1.2 0.5]);
      | plot([0.5 0],[0.5 -0.2]);
      | plot([-0.5 0],[0.5 -0.2]);
      | % Plot points to set plotting range
      | color('white');plot(1.3,1.3);plot(-1.3,-1.3)
      | color('black');
      | 
      | port_label('LConn',1,'A');
      | port_label('RConn',1,'B');
      | port_label('RConn',2,'T');
  Expansion Valve : Subsystem
      mask Display:
      | % Colored patches
      | patch([-1 -1 0],[0.5 -0.5 0],[1;0.4;0.4]);
      | patch([1 1 0],[0.5 -0.5 0],[0.4;0.4;1]);
      | % Valve
      | plot([1 1],[0.5 -0.5]);
      | plot([-1 -1],[0.5 -0.5]);
      | plot([-1 1],[0.5 -0.5]);
      | plot([-1 1],[-0.5 0.5]);
      | % Arrow
      | patch([1.15*sin(-pi/4-0.01);1.15*sin(-pi/4+0.01);1*sin(3*pi/4-0.01);1*sin(3*pi/4+0.01)],[1.15*cos(-pi/4-0.01);1.15*cos(-pi/4+0.01);1*cos(3*pi/4-0.01);1*cos(3*pi/4+0.01)],[0;0;0])
      | patch([0.8*sin(3*pi/4+0.07);1.15*sin(3*pi/4+0.00);1.15*sin(3*pi/4-0.00);0.8*sin(3*pi/4-0.07)],[0.8*cos(3*pi/4+0.07);1.15*cos(3*pi/4+0.00);1.15*cos(3*pi/4-0.00);0.8*cos(3*pi/4-0.07)],[0;0;0])
      | % Plot outer points to set plot range
      | color('white'); plot(-1.3,0); plot(1.3,0);
      | color('black');
      | port_label('LConn',1,'A');
      | port_label('RConn',1,'B');
  Fluid Properties : refrigeration_lib/Fluid Properties  p_TLU=p_TLU MPa  u_TLU=u_TLU kJ/kg  v_TLU=v_TLU m^3/kg  T_TLU=T_TLU K  mu_TLU=mu_TLU s*uPa  k_TLU=k_TLU W/(m*K)  Pr_TLU=Pr_TLU  u_liq=u_sat(:,1) kJ/kg  u_vap=u_sat(:,2) kJ/kg
      settings: InternalSimscapePortConfiguration="{\"Bottom\":[],\"Left\":[],\"Right\":[{\"id\":\"A\",\"label\":\"\",\"type\":\"refrigeration.refrigeration\"}],\"Top\":[]}"
  Mux : Mux  Inputs=2
  Plot Properties : Subsystem
      settings: OpenFcn=plotFluidProperties()
      mask Display: disp('Plot Fluid\nProperties');
  Refrigerator Compartment : Subsystem
      mask Display:
      | % Color
      | patch([sin(0:0.1:1*pi)*0.25+0.4 sin(pi:0.1:2*pi)*0.25-0.4],[cos(0:0.1:1*pi) cos(pi:0.1:2*pi)],[0.70;0.90;1]);
      | % Outer rounded rectangle
      | plot(sin(pi:0.1:2*pi)*0.25-0.4,cos(pi:0.1:2*pi));
      | plot(sin(0:0.1:1*pi)*0.25+0.4,cos(0:0.1:1*pi));
      | plot(sin(pi:0.1:2*pi)*0.25-0.4,cos(pi:0.1:2*pi));
      | plot([-0.4 0.4],[1 1]);
      | plot([-0.4 0.4],[-1 -1]);
      | % Outer points to set size of plot range
      | color('white');plot(0.8660,0.8660);plot(-0.8660,-0.8660)
      | color('black');
      | % Snowflake
      | plot([0 0],[0.8 -0.8]);
      | plot([0 0.1],[0.5 0.7]);
      | plot([0 -0.1],[0.5 0.7]);
      | plot([0 0.1],[-0.5 -0.7]);
      | plot([0 -0.1],[-0.5 -0.7]);
      | plot(0.3*sin([pi/3 4*pi/3]),1*cos([pi/3 4*pi/3]));
      | plot([0.22*sin(pi/3) 0.25*sin(pi/4)],[0.7*cos(pi/3) 0.84*cos(pi/4)]);
      | plot([0.22*sin(pi/3) 0.25*sin(pi/2)],[0.7*cos(pi/3) 0.325*cos(pi/4)]);
      | plot([0.22*sin(pi/3) 0.25*sin(pi/4)],[-0.7*cos(pi/3) -0.84*cos(pi/4)]);
      | plot([0.22*sin(pi/3) 0.25*sin(pi/2)],[-0.7*cos(pi/3) -0.325*cos(pi/4)]);
      | plot(-0.3*sin([pi/3 4*pi/3]),1*cos([pi/3 4*pi/3]));
      | plot([-0.22*sin(pi/3) -0.25*sin(pi/4)],[0.7*cos(pi/3) 0.84*cos(pi/4)]);
      | plot([-0.22*sin(pi/3) -0.25*sin(pi/2)],[0.7*cos(pi/3) 0.325*cos(pi/4)]);
      | plot([-0.22*sin(pi/3) -0.25*sin(pi/4)],[-0.7*cos(pi/3) -0.84*cos(pi/4)]);
      | plot([-0.22*sin(pi/3) -0.25*sin(pi/2)],[-0.7*cos(pi/3) -0.325*cos(pi/4)]);
      | plot([0 0.1],[-0.5 -0.7]);
      | plot([0 -0.1],[-0.5 -0.7]);
      | % Labels
      | port_label('LConn',1,'T');
      | port_label('output',1,'S');
  Refrigerator Temperature : Scope
  Sum1 : Sum  Inputs=|-+
  Target Refrigerator Temperature : Constant  Value=target_temperature
  Air : PMIOPort  Side=Left
  wires:
  Control/1(On) -> Compressor/1(On)
  Refrigerator Compartment/1(S) -> Mux/2, Sum1/2
  Target Refrigerator Temperature/1 -> Sum1/1, Mux/1
  Mux/1 -> Refrigerator Temperature/1
  Sum1/1 -> Control/1(Err)
  connections:
  Expansion Valve/RConn1 -- Fluid Properties/RConn1 -- Evaporator/LConn1
  Environment/LConn1 -- Condenser/LConn1
  Evaporator/RConn2 -- Refrigerator Compartment/LConn1
  Compressor/LConn1 -- Evaporator/RConn1
  Condenser/LConn2 -- Expansion Valve/LConn1
  Compressor/RConn1 -- Condenser/RConn1
  Refrigerator Compartment/LConn2 -- Air/RConn1

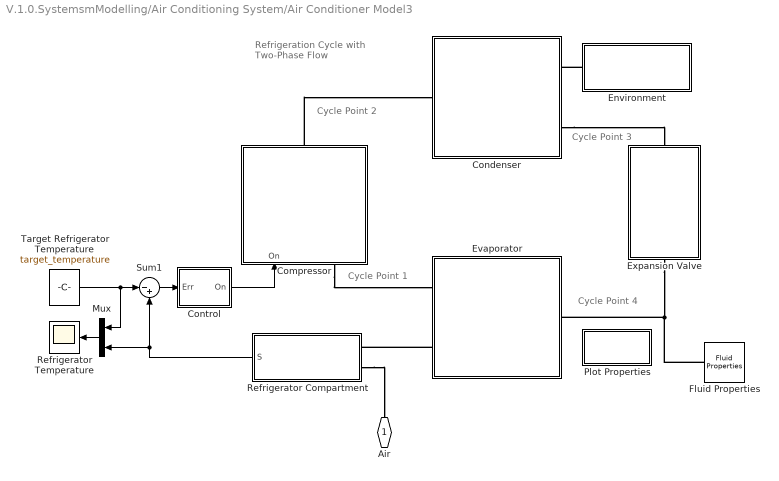
== system V.1.0.SystemsmModelling/Air Conditioning System/Air Conditioner Model3 ==
  note: Refrigeration Cycle
      | with Two-Phase Flow
  note: Cycle Point 1
  note: Cycle Point 3
  note: Cycle Point 2
  note: Cycle Point 4
  Compressor : Subsystem
      mask Display:
      | % Fading color
      | % Center to right
      | patch(sin(0.00*pi:0.05:1.10*pi),cos(0.00*pi:0.05:1.10*pi),[1;0.90;0.94]);
      | patch(sin(0.05*pi:0.05:0.95*pi),cos(0.05*pi:0.05:0.95*pi),[1;0.85;0.88]);
      | patch(sin(0.10*pi:0.05:0.90*pi),cos(0.10*pi:0.05:0.90*pi),[1;0.80;0.82]);
      | patch(sin(0.15*pi:0.05:0.85*pi),cos(0.15*pi:0.05:0.85*pi),[1;0.75;0.76]);
      | patch(sin(0.20*pi:0.05:0.80*pi),cos(0.20*pi:0.05:0.80*pi),[1;0.70;0.70]);
      | % Center to left
      | patch(sin(1.00*pi:0.05:2.00*pi),cos(1.00*pi:0.05:2.00*pi),[0.94;0.90;1]);
      | patch(sin(1.05*pi:0.05:1.95*pi),cos(1.05*pi:0.05:1.95*pi),[0.88;0.90;1]);
      | patch(sin(1.10*pi:0.05:1.90*pi),cos(1.10*pi:0.05:1.90*pi),[0.82;0.90;1]);
      | patch(sin(1.15*pi:0.05:1.85*pi),cos(1.15*pi:0.05:1.85*pi),[0.76;0.90;1]);
      | patch(sin(1.20*pi:0.05:1.80*pi),cos(1.20*pi:0.05:1.80*pi),[0.70;0.90;1]);
      | % Circle
      | plot(sin(0:0.1:2.2*pi),cos(0:0.1:2.2*pi));
      | % Angled lines
      | plot(sin([-0.6*pi/3 3.6*pi/8]),cos([-0.6*pi/3 3.6*pi/8]));
      | plot(sin([-0.6*pi/3 3.6*pi/8]),-cos([-0.6*pi/3 3.6*pi/8]));
      | plot(1.15*sin([-pi/4 3*pi/4]),1.15*cos([-pi/4 3*pi/4]));
      | % Arrow
      | patch([1.15*sin(-pi/4)+0.01;1.15*sin(3*pi/4)+0.01;1.15*sin(3*pi/4)-0.01;1.15*sin(-pi/4)-0.01],[1.15*cos(-pi/4)+0.01;1.15*cos(3*pi/4)+0.01;1.15*cos(3*pi/4)-0.01;1.15*cos(-pi/4)-0.01],[0;0;0])
      | patch([0.8*sin(3*pi/4)+0.05;1.15*sin(3*pi/4)+0.00;1.15*sin(3*pi/4)-0.00;0.8*sin(3*pi/4)-0.05],[0.8*cos(3*pi/4)+0.05;1.15*cos(3*pi/4)+0.00;1.15*cos(3*pi/4)-0.00;0.8*cos(3*pi/4)-0.05],[0;0;0])
      | % Points to set range for plotting area
      | color('white');plot(1.3,1.3);plot(-1.3,-1.3)
      | color('black');
      | 
      | port_label('LConn',1,'A');
      | port_label('RConn',1,'B');
      | port_label('input',1,'On');
  Condenser : Subsystem
      mask Display:
      | % Colored patches
      | % Center to right
      | patch(sin(0.0*pi:0.05:1.1*pi),cos(0.0*pi:0.05:1.1*pi),[1;0.58;0.58]);
      | patch(sin(0.1*pi:0.05:0.9*pi),cos(0.1*pi:0.05:0.9*pi),[1;0.64;0.64]);
      | patch(sin(0.2*pi:0.05:0.8*pi),cos(0.2*pi:0.05:0.8*pi),[1;0.70;0.70]);
      | % Center to left
      | patch(sin(1.0*pi:0.05:2.0*pi),cos(1.0*pi:0.05:2.0*pi),[1;0.52;0.52]);
      | patch(sin(1.1*pi:0.05:1.9*pi),cos(1.1*pi:0.05:1.9*pi),[1;0.46;0.46]);
      | patch(sin(1.2*pi:0.05:1.8*pi),cos(1.2*pi:0.05:1.8*pi),[1;0.40;0.40]);
      | % Circle
      | plot(sin(0:0.1:2.2*pi),cos(0:0.1:2.2*pi));
      | % 'M'
      | plot([0.5 0.5],[-1.2 0.5]);
      | plot([-0.5 -0.5],[-1.2 0.5]);
      | plot([0.5 0],[0.5 -0.2]);
      | plot([-0.5 0],[0.5 -0.2]);
      | % Plot points to set plot range
      | color('white');plot(1.3,1.3);plot(-1.3,-1.3)
      | color('black');
      | 
      | port_label('RConn',1,'A');
      | port_label('LConn',1,'T');
      | port_label('LConn',2,'B');
  Control : Subsystem
  Environment : Subsystem
      mask Display:
      | % Colored patch
      | patch([sin(0:0.1:1*pi)*0.25+0.4 sin(pi:0.1:2*pi)*0.25-0.4],[cos(0:0.1:1*pi) cos(pi:0.1:2*pi)],[1;0.9;0.9]);
      | % Outer rounded rectangle
      | plot(sin(0:0.1:1*pi)*0.25+0.4,cos(0:0.1:1*pi));
      | plot(sin(pi:0.1:2*pi)*0.25-0.4,cos(pi:0.1:2*pi));
      | plot([-0.4 0.4],[1 1]);
      | plot([-0.4 0.4],[-1 -1]);
      | % House frame
      | plot([-0.3 -0.3],[-0.866,0.866*0.2])
      | plot([0.3 0.3],[-0.866,0.866*0.2])
      | plot([0.3 0],[0.866*0.2, 0.866])
      | plot([-0.3 0],[0.866*0.2, 0.866])
      | plot([-0.3 0.3],[-0.866 -0.866])
      | plot([-0.3 0.3],[0.866 0.866]*0.2)
      | plot([-0.2 -0.04],[0.866 0.866]*0)
      | % Window
      | plot([-0.2 -0.04],[-1 -1]*0.2)
      | plot([-0.2 -0.04],[-1 -1]*0.4)
      | plot([-0.2 -0.2],[0 -0.4])
      | plot([-0.12 -0.12],[0 -0.4])
      | plot([-0.04 -0.04],[0 -0.4])
      | % Door
      | plot([0.05 0.05],[-0.866 -0.2])
      | plot([0.18 0.18],[-0.866 -0.2])
      | plot([0.05 0.18],[-0.2 -0.2])
      | patch([0.12 0.15 0.12 0.15],[-0.5 -0.5 -0.54 -0.54],[0;0;0])
      | % Outer boundary (so plot labels are visible)
      | color('white');plot(0.8660,0.8660);plot(-0.8660,-0.8660)
      | color('black');
      | port_label('LConn',1,'T');
  Evaporator : Subsystem
      mask Display:
      | % Fading color
      | % Center to right
      | patch(sin(0.00*pi:0.05:1.10*pi),cos(0.00*pi:0.05:1.10*pi),[0.58;0.70;1]);
      | patch(sin(0.05*pi:0.05:0.95*pi),cos(0.05*pi:0.05:0.95*pi),[0.63;0.75;1]);
      | patch(sin(0.10*pi:0.05:0.90*pi),cos(0.10*pi:0.05:0.90*pi),[0.66;0.80;1]);
      | patch(sin(0.15*pi:0.05:0.85*pi),cos(0.15*pi:0.05:0.85*pi),[0.69;0.85;1]);
      | patch(sin(0.20*pi:0.05:0.80*pi),cos(0.20*pi:0.05:0.80*pi),[0.70;0.90;1]);
      | % Center to left
      | patch(sin(1.00*pi:0.05:2.00*pi),cos(1.00*pi:0.05:2.00*pi),[0.52;0.60;1]);
      | patch(sin(1.05*pi:0.05:1.95*pi),cos(1.05*pi:0.05:1.95*pi),[0.49;0.55;1]);
      | patch(sin(1.10*pi:0.05:1.90*pi),cos(1.10*pi:0.05:1.90*pi),[0.46;0.50;1]);
      | patch(sin(1.15*pi:0.05:1.85*pi),cos(1.15*pi:0.05:1.85*pi),[0.43;0.45;1]);
      | patch(sin(1.20*pi:0.05:1.80*pi),cos(1.20*pi:0.05:1.80*pi),[0.40;0.40;1]);
      | % Circle
      | plot(sin(0:0.1:2.2*pi),cos(0:0.1:2.2*pi));
      | % 'M'
      | plot([0.5 0.5],[-1.2 0.5]);
      | plot([-0.5 -0.5],[-1.2 0.5]);
      | plot([0.5 0],[0.5 -0.2]);
      | plot([-0.5 0],[0.5 -0.2]);
      | % Plot points to set plotting range
      | color('white');plot(1.3,1.3);plot(-1.3,-1.3)
      | color('black');
      | 
      | port_label('LConn',1,'A');
      | port_label('RConn',1,'B');
      | port_label('RConn',2,'T');
  Expansion Valve : Subsystem
      mask Display:
      | % Colored patches
      | patch([-1 -1 0],[0.5 -0.5 0],[1;0.4;0.4]);
      | patch([1 1 0],[0.5 -0.5 0],[0.4;0.4;1]);
      | % Valve
      | plot([1 1],[0.5 -0.5]);
      | plot([-1 -1],[0.5 -0.5]);
      | plot([-1 1],[0.5 -0.5]);
      | plot([-1 1],[-0.5 0.5]);
      | % Arrow
      | patch([1.15*sin(-pi/4-0.01);1.15*sin(-pi/4+0.01);1*sin(3*pi/4-0.01);1*sin(3*pi/4+0.01)],[1.15*cos(-pi/4-0.01);1.15*cos(-pi/4+0.01);1*cos(3*pi/4-0.01);1*cos(3*pi/4+0.01)],[0;0;0])
      | patch([0.8*sin(3*pi/4+0.07);1.15*sin(3*pi/4+0.00);1.15*sin(3*pi/4-0.00);0.8*sin(3*pi/4-0.07)],[0.8*cos(3*pi/4+0.07);1.15*cos(3*pi/4+0.00);1.15*cos(3*pi/4-0.00);0.8*cos(3*pi/4-0.07)],[0;0;0])
      | % Plot outer points to set plot range
      | color('white'); plot(-1.3,0); plot(1.3,0);
      | color('black');
      | port_label('LConn',1,'A');
      | port_label('RConn',1,'B');
  Fluid Properties : refrigeration_lib/Fluid Properties  p_TLU=p_TLU MPa  u_TLU=u_TLU kJ/kg  v_TLU=v_TLU m^3/kg  T_TLU=T_TLU K  mu_TLU=mu_TLU s*uPa  k_TLU=k_TLU W/(m*K)  Pr_TLU=Pr_TLU  u_liq=u_sat(:,1) kJ/kg  u_vap=u_sat(:,2) kJ/kg
      settings: InternalSimscapePortConfiguration="{\"Bottom\":[],\"Left\":[],\"Right\":[{\"id\":\"A\",\"label\":\"\",\"type\":\"refrigeration.refrigeration\"}],\"Top\":[]}"
  Mux : Mux  Inputs=2
  Plot Properties : Subsystem
      settings: OpenFcn=plotFluidProperties()
      mask Display: disp('Plot Fluid\nProperties');
  Refrigerator Compartment : Subsystem
      mask Display:
      | % Color
      | patch([sin(0:0.1:1*pi)*0.25+0.4 sin(pi:0.1:2*pi)*0.25-0.4],[cos(0:0.1:1*pi) cos(pi:0.1:2*pi)],[0.70;0.90;1]);
      | % Outer rounded rectangle
      | plot(sin(pi:0.1:2*pi)*0.25-0.4,cos(pi:0.1:2*pi));
      | plot(sin(0:0.1:1*pi)*0.25+0.4,cos(0:0.1:1*pi));
      | plot(sin(pi:0.1:2*pi)*0.25-0.4,cos(pi:0.1:2*pi));
      | plot([-0.4 0.4],[1 1]);
      | plot([-0.4 0.4],[-1 -1]);
      | % Outer points to set size of plot range
      | color('white');plot(0.8660,0.8660);plot(-0.8660,-0.8660)
      | color('black');
      | % Snowflake
      | plot([0 0],[0.8 -0.8]);
      | plot([0 0.1],[0.5 0.7]);
      | plot([0 -0.1],[0.5 0.7]);
      | plot([0 0.1],[-0.5 -0.7]);
      | plot([0 -0.1],[-0.5 -0.7]);
      | plot(0.3*sin([pi/3 4*pi/3]),1*cos([pi/3 4*pi/3]));
      | plot([0.22*sin(pi/3) 0.25*sin(pi/4)],[0.7*cos(pi/3) 0.84*cos(pi/4)]);
      | plot([0.22*sin(pi/3) 0.25*sin(pi/2)],[0.7*cos(pi/3) 0.325*cos(pi/4)]);
      | plot([0.22*sin(pi/3) 0.25*sin(pi/4)],[-0.7*cos(pi/3) -0.84*cos(pi/4)]);
      | plot([0.22*sin(pi/3) 0.25*sin(pi/2)],[-0.7*cos(pi/3) -0.325*cos(pi/4)]);
      | plot(-0.3*sin([pi/3 4*pi/3]),1*cos([pi/3 4*pi/3]));
      | plot([-0.22*sin(pi/3) -0.25*sin(pi/4)],[0.7*cos(pi/3) 0.84*cos(pi/4)]);
      | plot([-0.22*sin(pi/3) -0.25*sin(pi/2)],[0.7*cos(pi/3) 0.325*cos(pi/4)]);
      | plot([-0.22*sin(pi/3) -0.25*sin(pi/4)],[-0.7*cos(pi/3) -0.84*cos(pi/4)]);
      | plot([-0.22*sin(pi/3) -0.25*sin(pi/2)],[-0.7*cos(pi/3) -0.325*cos(pi/4)]);
      | plot([0 0.1],[-0.5 -0.7]);
      | plot([0 -0.1],[-0.5 -0.7]);
      | % Labels
      | port_label('LConn',1,'T');
      | port_label('output',1,'S');
  Refrigerator Temperature : Scope
  Sum1 : Sum  Inputs=|-+
  Target Refrigerator Temperature : Constant  Value=target_temperature
  Air : PMIOPort  Side=Left
  wires:
  Control/1(On) -> Compressor/1(On)
  Refrigerator Compartment/1(S) -> Mux/2, Sum1/2
  Target Refrigerator Temperature/1 -> Sum1/1, Mux/1
  Mux/1 -> Refrigerator Temperature/1
  Sum1/1 -> Control/1(Err)
  connections:
  Expansion Valve/RConn1 -- Fluid Properties/RConn1 -- Evaporator/LConn1
  Environment/LConn1 -- Condenser/LConn1
  Evaporator/RConn2 -- Refrigerator Compartment/LConn1
  Compressor/LConn1 -- Evaporator/RConn1
  Condenser/LConn2 -- Expansion Valve/LConn1
  Compressor/RConn1 -- Condenser/RConn1
  Refrigerator Compartment/LConn2 -- Air/RConn1
